simulink model "B64CostaTest"  (R2022a)
settings: Solver=VariableStepAuto  StartTime=0.0  StopTime=40  RelTol=1e-4  AbsTol=1e-4
values from neighbouring files (symbols this model uses):
  AinfK_h_B64a = -23    [B64.m]
  AinfK_h_B64s = -23    [B64.m]
  AinfK_p_B64a = 1.0    (= 1)    [B64.m]
  AinfK_p_B64s = 1.0    (= 1)    [B64.m]
  AinfK_s_B64a = 9.0    (= 9)    [B64.m]
  AinfK_s_B64s = 9.0    (= 9)    [B64.m]
  AinfKpp_h_B64s = -50    [B64.m]
  AinfKpp_p_B64s = 1.0    (= 1)    [B64.m]
  AinfKpp_s_B64s = 1.0    (= 1)    [B64.m]
  AinfNa_h_B64a = -37    [B64.m]
  AinfNa_h_B64s = -37    [B64.m]
  AinfNa_p_B64a = 1.0    (= 1)    [B64.m]
  AinfNa_p_B64s = 1.0    (= 1)    [B64.m]
  AinfNa_s_B64a = 5.0    (= 5)    [B64.m]
  AinfNa_s_B64s = 5.0    (= 5)    [B64.m]
  AinfNapp_h_B64s = -50    [B64.m]
  AinfNapp_p_B64s = 1.0    (= 1)    [B64.m]
  AinfNapp_s_B64s = 1.0    (= 1)    [B64.m]
  AK_B64a_0 = 0.5    [B64.m]
  AK_B64s_0 = 0.5    [B64.m]
  AKpp_B64s_0 = 0.5    [B64.m]
  ANa_B64a_0 = 0.5    [B64.m]
  ANa_B64s_0 = 0.5    [B64.m]
  ANapp_B64s_0 = 0.5    [B64.m]
  BinfNa_h_B64a = -43.0    (= -43)    [B64.m]
  BinfNa_h_B64s = -43.0    (= -43)    [B64.m]
  BinfNa_p_B64a = 1.0    (= 1)    [B64.m]
  BinfNa_p_B64s = 1.0    (= 1)    [B64.m]
  BinfNa_s_B64a = 5.0    (= 5)    [B64.m]
  BinfNa_s_B64s = 5.0    (= 5)    [B64.m]
  BNa_B64a_0 = 0.5    [B64.m]
  BNa_B64s_0 = 0.5    [B64.m]
  Cm_B64a = 0.01    [B64.m]
  Cm_B64s = 0.01    [B64.m]
  EK_B64a = -70    [B64.m]
  EK_B64s = -80    [B64.m]
  EKpp_B64s = -70    [B64.m]
  EL_B64a = -60    [B64.m]
  EL_B64s = -60    [B64.m]
  ENa_B64a = 30    [B64.m]
  ENa_B64s = 30    [B64.m]
  ENapp_B64s = 30    [B64.m]
  gec_B64a2B64s = 0.25    [B64.m]
  gec_B64s2B64a = 0.25    [B64.m]
  gK_B64a = 14    [B64.m]
  gK_B64s = 1.2    [B64.m]
  gKpp_B64s = 0.35    [B64.m]
  gL_B64a = 0.1    [B64.m]
  gL_B64s = 0.1    [B64.m]
  gNa_B64a = 25    [B64.m]
  gNa_B64s = 2.5    [B64.m]
  gNapp_B64s = 0.1    [B64.m]
  pK_B64a = 4    [B64.m]
  pK_B64s = 4    [B64.m]
  pKpp_B64s = 1    [B64.m]
  pNa_B64a = 3    [B64.m]
  pNa_B64s = 3    [B64.m]
  pNapp_B64s = 1    [B64.m]
  RK_B64a = 0    [B64.m]
  RK_B64s = 0    [B64.m]
  RKpp_B64s = 0    [B64.m]
  RL_B64a = 0    [B64.m]
  RL_B64s = 0    [B64.m]
  RNa_B64a = 0    [B64.m]
  RNa_B64s = 0    [B64.m]
  RNapp_B64s = 0    [B64.m]
  spikedur_B64a = 0.003    [B64.m]
  tAK_h_B64a = -8.0    (= -8)    [B64.m]
  tAK_h_B64s = -8.0    (= -8)    [B64.m]
  tAK_p_B64a = 1.0    (= 1)    [B64.m]
  tAK_p_B64s = 1.0    (= 1)    [B64.m]
  tAK_s_B64a = 10.0    (= 10)    [B64.m]
  tAK_s_B64s = 10.0    (= 10)    [B64.m]
  tAK_tmax_B64a = 0.04    [B64.m]
  tAK_tmax_B64s = 0.04    [B64.m]
  tAK_tmin_B64a = 0.004    [B64.m]
  tAK_tmin_B64s = 0.004    [B64.m]
  tAKpp_t_B64s = 4    [B64.m]
  tANa_h_B64a = -43    [B64.m]
  tANa_h_B64s = -43    [B64.m]
  tANa_p_B64a = 1.0    (= 1)    [B64.m]
  tANa_p_B64s = 1.0    (= 1)    [B64.m]
  tANa_s_B64a = 4.0    (= 4)    [B64.m]
  tANa_s_B64s = 4.0    (= 4)    [B64.m]
  tANa_tmax_B64a = 0.006    [B64.m]
  tANa_tmax_B64s = 0.006    [B64.m]
  tANa_tmin_B64a = 0.001    [B64.m]
  tANa_tmin_B64s = 0.001    [B64.m]
  tANapp_t_B64s = 0.1    [B64.m]
  tBNa_h_B64a = -38    [B64.m]
  tBNa_h_B64s = -38    [B64.m]
  tBNa_p_B64a = 1.0    (= 1)    [B64.m]
  tBNa_p_B64s = 1.0    (= 1)    [B64.m]
  tBNa_s_B64a = 10.0    (= 10)    [B64.m]
  tBNa_s_B64s = 10.0    (= 10)    [B64.m]
  tBNa_tmax_B64a = 0.02    [B64.m]
  tBNa_tmax_B64s = 0.02    [B64.m]
  tBNa_tmin_B64a = 0.005    [B64.m]
  tBNa_tmin_B64s = 0.005    [B64.m]
  V_B64a_0 = -60    [B64.m]
  V_B64s_0 = -60    [B64.m]
undefined symbols (not defined in the file or in its folder): Iapp
libraries: simulink x1
settings Model: Creator=liyan  LastModifiedBy=liyan

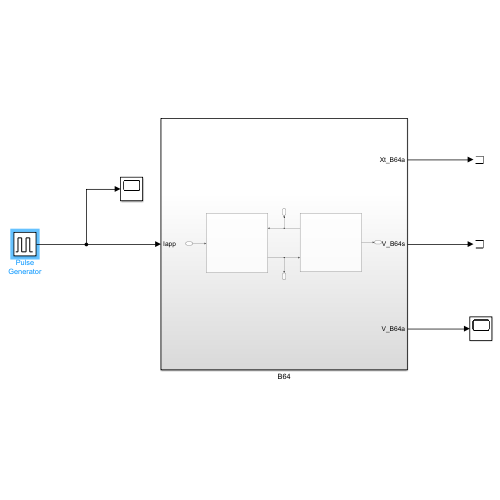
[thumbnail: Simulink's stored preview of the top-level diagram]
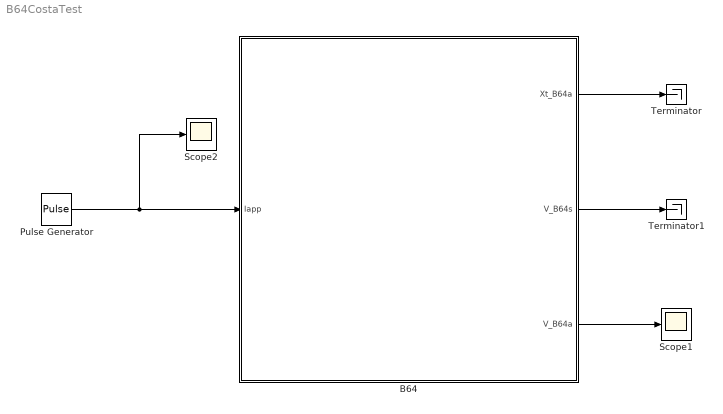
== system B64CostaTest ==
  B64 : Subsystem
  Pulse Generator : DiscretePulseGenerator  PulseType=Time based  Amplitude=Iapp  Period=40  PulseWidth=0.3/40*100  PhaseDelay=30
  Scope1 : Scope
  Scope2 : Scope
  Terminator : Terminator
  Terminator1 : Terminator
  wires:
  Pulse Generator/1 -> B64/1(Iapp), Scope2/1
  B64/2(V_B64s) -> Terminator1/1
  B64/3(V_B64a) -> Scope1/1
  B64/1(Xt_B64a) -> Terminator/1

== system B64CostaTest/B64 ==
  Iapp : Inport
  Axon : Subsystem
      settings: PortSchema="{\"entries\":[{\"content\":{\"sides\":[{\"content\":{\"connectorIds\":[\"In1\",\"Out2\"]},\"type\":\"ConnectorPlacement.EquallySpacedRectSide\",\"uuid\":\"40bd10fa-ed99-4b6a-86ee-aa667b2fa219\"},{\"content\":{\"connectorIds\":[\"Out1\"],\"side\":\"RIGHT\"},\"type\":\"ConnectorPlacement.EquallySpacedRectSide\",\"uuid\":\"a431bac5-795f-4390-8885-144606cfe2c6\"},{\"content\":{\"connectorIds\":[],\"side\":\"TOP\"},\"type\":\"ConnectorPlacement.EquallySpacedRectSide\",\"uuid\":\"7e20a892-1662-4491-8c8d-274d49de163b\"},{\"content\":{\"connectorIds\":[],\"side\":\"BOTTOM\"},\"type\":\"ConnectorPlacement.EquallySpacedRectSide\",\"uuid\":\"ab3dc877-3a3e-482a-aafe-64d6d0026420\"}]},\"type\":\"ConnectorPlacement.EquallySpacedConnector\",\"uuid\":\"01fbcc32-18b1-446e-a5b1-3660a779301b\"}],\"packageUris\":[\"http://schema.mathworks.com/mf0/Connector/R2020b\"],\"version\":\"1.0\"}"
  Soma : Subsystem
      settings: PortSchema="{\"entries\":[{\"content\":{\"sides\":[{\"content\":{\"connectorIds\":[\"In1\"]},\"type\":\"ConnectorPlacement.EquallySpacedRectSide\",\"uuid\":\"61f6e0bf-b055-4ffe-aeac-0536888a11b7\"},{\"content\":{\"connectorIds\":[\"Out1\",\"In2\"],\"side\":\"RIGHT\"},\"type\":\"ConnectorPlacement.EquallySpacedRectSide\",\"uuid\":\"fd31abd7-219d-468a-b386-105a5f18ecba\"},{\"content\":{\"connectorIds\":[],\"side\":\"TOP\"},\"type\":\"ConnectorPlacement.EquallySpacedRectSide\",\"uuid\":\"61248356-ebfa-4703-87fc-ac9a699c85cb\"},{\"content\":{\"connectorIds\":[],\"side\":\"BOTTOM\"},\"type\":\"ConnectorPlacement.EquallySpacedRectSide\",\"uuid\":\"824f436a-a50d-431e-bf8e-5e4435a63c06\"}]},\"type\":\"ConnectorPlacement.EquallySpacedConnector\",\"uuid\":\"04bfac00-4a5c-4c95-bc84-ba6035aba6c8\"}],\"packageUris\":[\"http://schema.mathworks.com/mf0/Connector/R2020b\"],\"version\":\"1.0\"}"
  Xt_B64a : Outport
  V_B64s : Outport  Port=2
  V_B64a : Outport  Port=3
  wires:
  Axon/2(V_B64a) -> V_B64a/1, Soma/2(V_B64a)
  Soma/1(V_B64s) -> V_B64s/1, Axon/1(V_B64s)
  Axon/1(Xt_B64a) -> Xt_B64a/1
  Iapp/1 -> Soma/1(Iapp)

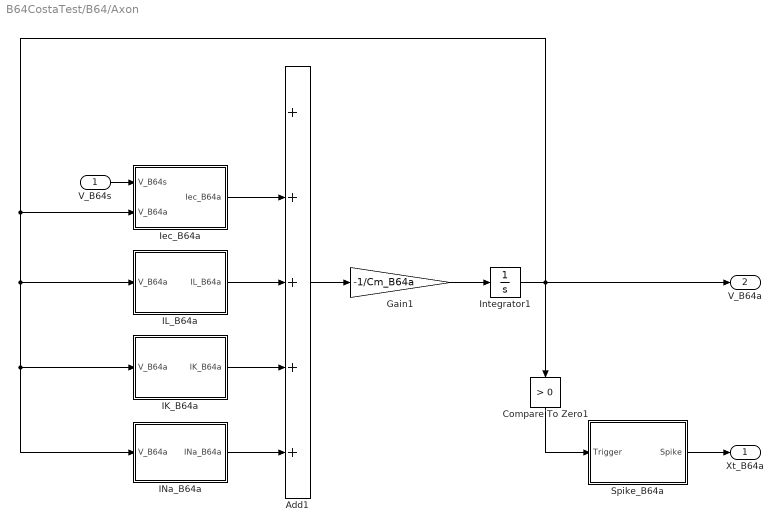
== system B64CostaTest/B64/Axon ==
  V_B64s : Inport
  Add1 : Sum  Inputs=+++++
  Compare To Zero1 : simulink/Logic and Bit Operations/Compare To Zero  relop=>  OutDataTypeStr=boolean
  Gain1 : Gain  Gain=-1/Cm_B64a
  IK_B64a : Subsystem
  IL_B64a : Subsystem
  INa_B64a : Subsystem
  Iec_B64a : Subsystem
  Integrator1 : Integrator  InitialCondition=V_B64a_0
  Spike_B64a : Subsystem
  Xt_B64a : Outport
  V_B64a : Outport  Port=2
  wires:
  Add1/1 -> Gain1/1
  Gain1/1 -> Integrator1/1
  Integrator1/1 -> Iec_B64a/2(V_B64a), IL_B64a/1(V_B64a), IK_B64a/1(V_B64a), INa_B64a/1(V_B64a), Compare To Zero1/1, V_B64a/1
  V_B64s/1 -> Iec_B64a/1(V_B64s)
  Compare To Zero1/1 -> Spike_B64a/1(Trigger)
  Spike_B64a/1(Spike) -> Xt_B64a/1
  INa_B64a/1(INa_B64a) -> Add1/5
  IK_B64a/1(IK_B64a) -> Add1/4
  IL_B64a/1(IL_B64a) -> Add1/3
  Iec_B64a/1(Iec_B64a) -> Add1/2

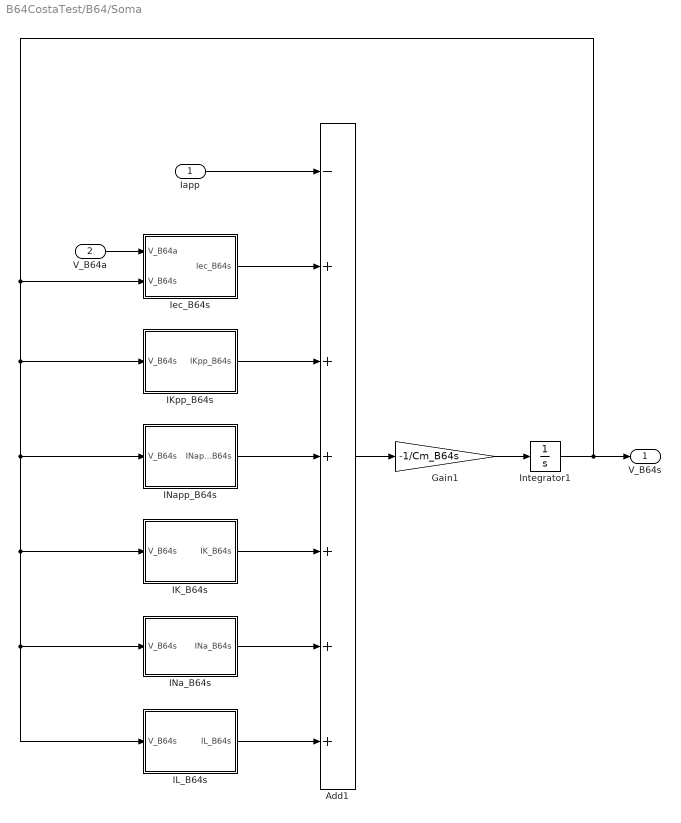
== system B64CostaTest/B64/Soma ==
  Iapp : Inport
  V_B64a : Inport  Port=2
  Add1 : Sum  Inputs=-++++++
  Gain1 : Gain  Gain=-1/Cm_B64s
  IK_B64s : Subsystem
  IKpp_B64s : Subsystem
  IL_B64s : Subsystem
  INa_B64s : Subsystem
  INapp_B64s : Subsystem
  Iec_B64s : Subsystem
  Integrator1 : Integrator  InitialCondition=V_B64s_0
  V_B64s : Outport
  wires:
  Add1/1 -> Gain1/1
  Gain1/1 -> Integrator1/1
  V_B64a/1 -> Iec_B64s/1(V_B64a)
  IL_B64s/1(IL_B64s) -> Add1/7
  INa_B64s/1(INa_B64s) -> Add1/6
  IK_B64s/1(IK_B64s) -> Add1/5
  INapp_B64s/1(INapp_B64s) -> Add1/4
  IKpp_B64s/1(IKpp_B64s) -> Add1/3
  Iec_B64s/1(Iec_B64s) -> Add1/2
  Integrator1/1 -> V_B64s/1, IKpp_B64s/1(V_B64s), INapp_B64s/1(V_B64s), IK_B64s/1(V_B64s), INa_B64s/1(V_B64s), IL_B64s/1(V_B64s), Iec_B64s/2(V_B64s)
  Iapp/1 -> Add1/1

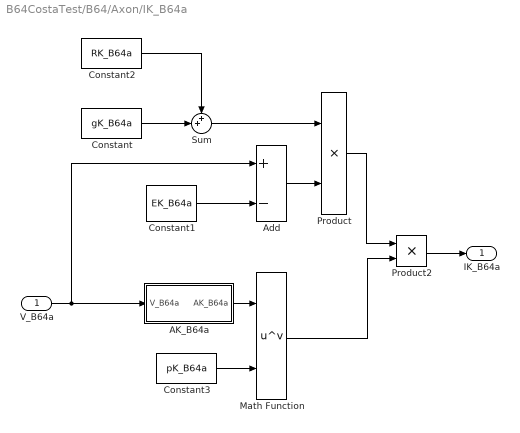
== system B64CostaTest/B64/Axon/IK_B64a ==
  V_B64a : Inport
  AK_B64a : Subsystem
  Add : Sum  Inputs=+-
  Constant : Constant  Value=gK_B64a
  Constant1 : Constant  Value=EK_B64a
  Constant2 : Constant  Value=RK_B64a
  Constant3 : Constant  Value=pK_B64a
  Math Function : Math  Operator=pow
  Product : Product
  Product2 : Product
  Sum : Sum  Inputs=++|
  IK_B64a : Outport
  wires:
  Add/1 -> Product/2
  Constant1/1 -> Add/2
  V_B64a/1 -> AK_B64a/1(V_B64a), Add/1
  Product/1 -> Product2/1
  Math Function/1 -> Product2/2
  Product2/1 -> IK_B64a/1
  Constant/1 -> Sum/2
  Sum/1 -> Product/1
  Constant2/1 -> Sum/1
  AK_B64a/1(AK_B64a) -> Math Function/1
  Constant3/1 -> Math Function/2

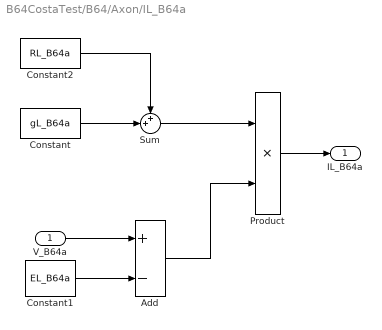
== system B64CostaTest/B64/Axon/IL_B64a ==
  V_B64a : Inport
  Add : Sum  Inputs=+-
  Constant : Constant  Value=gL_B64a
  Constant1 : Constant  Value=EL_B64a
  Constant2 : Constant  Value=RL_B64a
  Product : Product
  Sum : Sum  Inputs=++|
  IL_B64a : Outport
  wires:
  Constant1/1 -> Add/2
  V_B64a/1 -> Add/1
  Constant2/1 -> Sum/1
  Sum/1 -> Product/1
  Constant/1 -> Sum/2
  Add/1 -> Product/2
  Product/1 -> IL_B64a/1

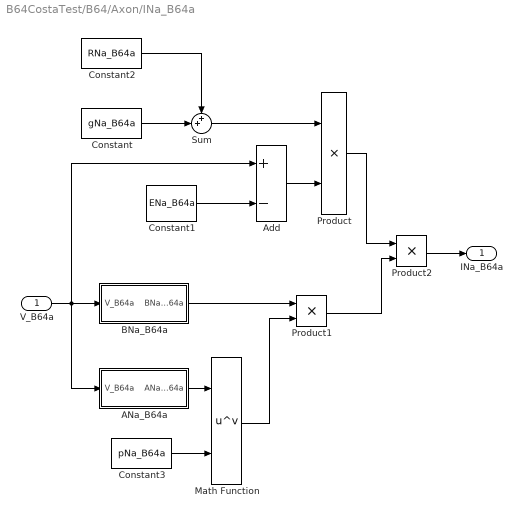
== system B64CostaTest/B64/Axon/INa_B64a ==
  V_B64a : Inport
  ANa_B64a : Subsystem
  Add : Sum  Inputs=+-
  BNa_B64a : Subsystem
  Constant : Constant  Value=gNa_B64a
  Constant1 : Constant  Value=ENa_B64a
  Constant2 : Constant  Value=RNa_B64a
  Constant3 : Constant  Value=pNa_B64a
  Math Function : Math  Operator=pow
  Product : Product
  Product1 : Product
  Product2 : Product
  Sum : Sum  Inputs=++|
  INa_B64a : Outport
  wires:
  Add/1 -> Product/2
  Constant1/1 -> Add/2
  V_B64a/1 -> ANa_B64a/1(V_B64a), BNa_B64a/1(V_B64a), Add/1
  Product/1 -> Product2/1
  Product1/1 -> Product2/2
  Product2/1 -> INa_B64a/1
  Constant/1 -> Sum/2
  Sum/1 -> Product/1
  Constant2/1 -> Sum/1
  ANa_B64a/1(ANa_B64a) -> Math Function/1
  Constant3/1 -> Math Function/2
  BNa_B64a/1(BNa_B64a) -> Product1/1
  Math Function/1 -> Product1/2

== system B64CostaTest/B64/Axon/Iec_B64a ==
  V_B64s : Inport
  V_B64a : Inport  Port=2
  Add : Sum  Inputs=-+
  Gain : Gain  Gain=gec_B64s2B64a
  Iec_B64a : Outport
  wires:
  Add/1 -> Gain/1
  V_B64s/1 -> Add/1
  V_B64a/1 -> Add/2
  Gain/1 -> Iec_B64a/1

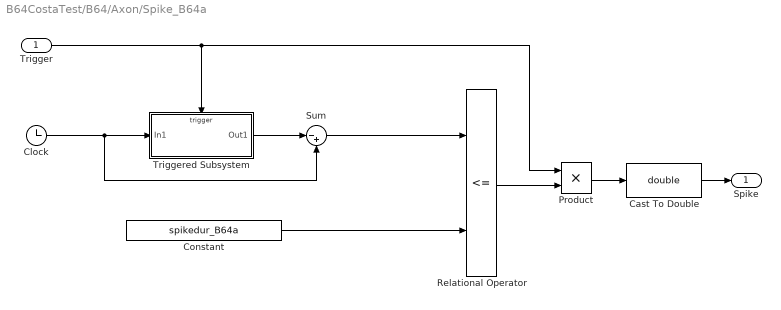
== system B64CostaTest/B64/Axon/Spike_B64a ==
  Trigger : Inport
  Cast To Double : DataTypeConversion  OutDataTypeStr=double  SaturateOnIntegerOverflow=off  RndMeth=Floor
  Clock : Clock
  Constant : Constant  Value=spikedur_B64a
  Product : Product
  Relational Operator : RelationalOperator  Operator=<=  OutDataTypeStr=boolean  RndMeth=Simplest  InputSameDT=off
  Sum : Sum  Inputs=|-+
  Triggered Subsystem : Subsystem  TreatAsAtomicUnit=on
  Spike : Outport
  wires:
  Clock/1 -> Sum/2, Triggered Subsystem/1(In1)
  Triggered Subsystem/1(Out1) -> Sum/1
  Constant/1 -> Relational Operator/2
  Trigger/1 -> Triggered Subsystem/Trigger, Product/1
  Sum/1 -> Relational Operator/1
  Relational Operator/1 -> Product/2
  Cast To Double/1 -> Spike/1
  Product/1 -> Cast To Double/1

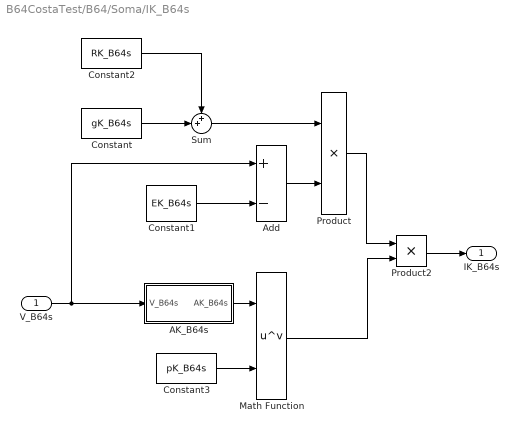
== system B64CostaTest/B64/Soma/IK_B64s ==
  V_B64s : Inport
  AK_B64s : Subsystem
  Add : Sum  Inputs=+-
  Constant : Constant  Value=gK_B64s
  Constant1 : Constant  Value=EK_B64s
  Constant2 : Constant  Value=RK_B64s
  Constant3 : Constant  Value=pK_B64s
  Math Function : Math  Operator=pow
  Product : Product
  Product2 : Product
  Sum : Sum  Inputs=++|
  IK_B64s : Outport
  wires:
  Add/1 -> Product/2
  Constant1/1 -> Add/2
  V_B64s/1 -> AK_B64s/1(V_B64s), Add/1
  Product/1 -> Product2/1
  Math Function/1 -> Product2/2
  Product2/1 -> IK_B64s/1
  Constant/1 -> Sum/2
  Sum/1 -> Product/1
  Constant2/1 -> Sum/1
  AK_B64s/1(AK_B64s) -> Math Function/1
  Constant3/1 -> Math Function/2

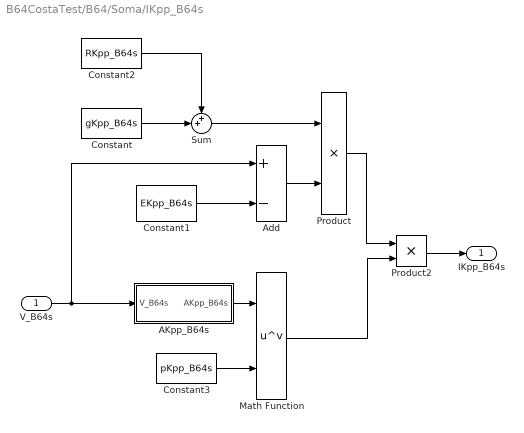
== system B64CostaTest/B64/Soma/IKpp_B64s ==
  V_B64s : Inport
  AKpp_B64s : Subsystem
  Add : Sum  Inputs=+-
  Constant : Constant  Value=gKpp_B64s
  Constant1 : Constant  Value=EKpp_B64s
  Constant2 : Constant  Value=RKpp_B64s
  Constant3 : Constant  Value=pKpp_B64s
  Math Function : Math  Operator=pow
  Product : Product
  Product2 : Product
  Sum : Sum  Inputs=++|
  IKpp_B64s : Outport
  wires:
  Add/1 -> Product/2
  Constant1/1 -> Add/2
  V_B64s/1 -> AKpp_B64s/1(V_B64s), Add/1
  Product/1 -> Product2/1
  Math Function/1 -> Product2/2
  Product2/1 -> IKpp_B64s/1
  Constant/1 -> Sum/2
  Sum/1 -> Product/1
  Constant2/1 -> Sum/1
  AKpp_B64s/1(AKpp_B64s) -> Math Function/1
  Constant3/1 -> Math Function/2

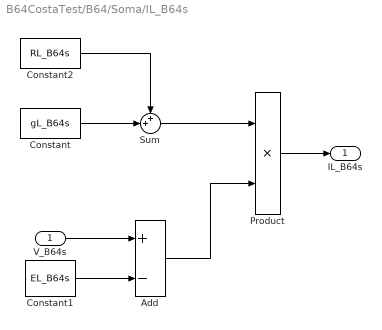
== system B64CostaTest/B64/Soma/IL_B64s ==
  V_B64s : Inport
  Add : Sum  Inputs=+-
  Constant : Constant  Value=gL_B64s
  Constant1 : Constant  Value=EL_B64s
  Constant2 : Constant  Value=RL_B64s
  Product : Product
  Sum : Sum  Inputs=++|
  IL_B64s : Outport
  wires:
  Constant1/1 -> Add/2
  V_B64s/1 -> Add/1
  Constant2/1 -> Sum/1
  Sum/1 -> Product/1
  Constant/1 -> Sum/2
  Add/1 -> Product/2
  Product/1 -> IL_B64s/1

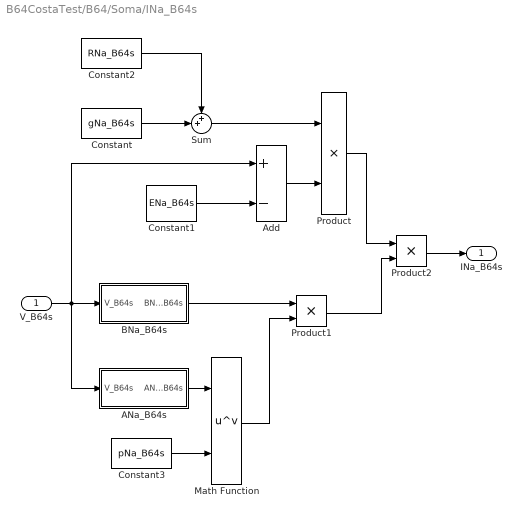
== system B64CostaTest/B64/Soma/INa_B64s ==
  V_B64s : Inport
  ANa_B64s : Subsystem
  Add : Sum  Inputs=+-
  BNa_B64s : Subsystem
  Constant : Constant  Value=gNa_B64s
  Constant1 : Constant  Value=ENa_B64s
  Constant2 : Constant  Value=RNa_B64s
  Constant3 : Constant  Value=pNa_B64s
  Math Function : Math  Operator=pow
  Product : Product
  Product1 : Product
  Product2 : Product
  Sum : Sum  Inputs=++|
  INa_B64s : Outport
  wires:
  Add/1 -> Product/2
  Constant1/1 -> Add/2
  V_B64s/1 -> ANa_B64s/1(V_B64s), BNa_B64s/1(V_B64s), Add/1
  Product/1 -> Product2/1
  Product1/1 -> Product2/2
  Product2/1 -> INa_B64s/1
  Constant/1 -> Sum/2
  Sum/1 -> Product/1
  Constant2/1 -> Sum/1
  ANa_B64s/1(ANa_B64s) -> Math Function/1
  Constant3/1 -> Math Function/2
  BNa_B64s/1(BNa_B64s) -> Product1/1
  Math Function/1 -> Product1/2

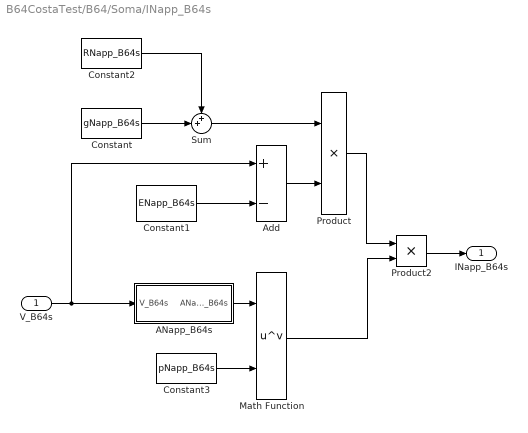
== system B64CostaTest/B64/Soma/INapp_B64s ==
  V_B64s : Inport
  ANapp_B64s : Subsystem
  Add : Sum  Inputs=+-
  Constant : Constant  Value=gNapp_B64s
  Constant1 : Constant  Value=ENapp_B64s
  Constant2 : Constant  Value=RNapp_B64s
  Constant3 : Constant  Value=pNapp_B64s
  Math Function : Math  Operator=pow
  Product : Product
  Product2 : Product
  Sum : Sum  Inputs=++|
  INapp_B64s : Outport
  wires:
  Add/1 -> Product/2
  Constant1/1 -> Add/2
  V_B64s/1 -> ANapp_B64s/1(V_B64s), Add/1
  Product/1 -> Product2/1
  Math Function/1 -> Product2/2
  Product2/1 -> INapp_B64s/1
  Constant/1 -> Sum/2
  Sum/1 -> Product/1
  Constant2/1 -> Sum/1
  ANapp_B64s/1(ANapp_B64s) -> Math Function/1
  Constant3/1 -> Math Function/2

== system B64CostaTest/B64/Soma/Iec_B64s ==
  V_B64a : Inport
  V_B64s : Inport  Port=2
  Add : Sum  Inputs=-+
  Gain : Gain  Gain=gec_B64a2B64s
  Iec_B64s : Outport
  wires:
  Add/1 -> Gain/1
  V_B64a/1 -> Add/1
  V_B64s/1 -> Add/2
  Gain/1 -> Iec_B64s/1

== system B64CostaTest/B64/Axon/IK_B64a/AK_B64a ==
  V_B64a : Inport
  AKinf_B64a : MATLABFcn  MATLABFcn=1/(1 + exp((AinfK_h_B64a - u(1))/AinfK_s_B64a))^AinfK_p_B64a
  Add1 : Sum  Inputs=-+
  Divide : Product  Inputs=*/
  Integrator1 : Integrator  InitialCondition=AK_B64a_0
  tauAK_B64a : MATLABFcn  MATLABFcn=tAK_tmin_B64a + (tAK_tmax_B64a - tAK_tmin_B64a)/(1 + exp((u(1) - tAK_h_B64a)/tAK_s_B64a))^tAK_p_B64a
  AK_B64a : Outport
  wires:
  tauAK_B64a/1 -> Divide/2
  Divide/1 -> Integrator1/1
  V_B64a/1 -> tauAK_B64a/1, AKinf_B64a/1
  Integrator1/1 -> Add1/1, AK_B64a/1
  Add1/1 -> Divide/1
  AKinf_B64a/1 -> Add1/2

== system B64CostaTest/B64/Axon/INa_B64a/ANa_B64a ==
  V_B64a : Inport
  ANainf_B64a : MATLABFcn  MATLABFcn=1/(1 + exp((AinfNa_h_B64a - u(1))/AinfNa_s_B64a))^AinfNa_p_B64a
  Add1 : Sum  Inputs=-+
  Divide : Product  Inputs=*/
  Integrator1 : Integrator  InitialCondition=ANa_B64a_0
  tauANa_B64a : MATLABFcn  MATLABFcn=tANa_tmin_B64a + (tANa_tmax_B64a - tANa_tmin_B64a)/(1 + exp((u(1) - tANa_h_B64a)/tANa_s_B64a))^tANa_p_B64a
  ANa_B64a : Outport
  wires:
  tauANa_B64a/1 -> Divide/2
  Divide/1 -> Integrator1/1
  V_B64a/1 -> tauANa_B64a/1, ANainf_B64a/1
  Integrator1/1 -> Add1/1, ANa_B64a/1
  Add1/1 -> Divide/1
  ANainf_B64a/1 -> Add1/2

== system B64CostaTest/B64/Axon/INa_B64a/BNa_B64a ==
  V_B64a : Inport
  Add1 : Sum  Inputs=-+
  BNainf_B64a : MATLABFcn  MATLABFcn=1/(1 + exp((u(1) - BinfNa_h_B64a)/BinfNa_s_B64a))^BinfNa_p_B64a
  Divide : Product  Inputs=*/
  Integrator1 : Integrator  InitialCondition=BNa_B64a_0
  tauBNa_B64a : MATLABFcn  MATLABFcn=tBNa_tmin_B64a + (tBNa_tmax_B64a - tBNa_tmin_B64a)/(1 + exp((u(1) - tBNa_h_B64a)/tBNa_s_B64a))^tBNa_p_B64a
  BNa_B64a : Outport
  wires:
  tauBNa_B64a/1 -> Divide/2
  Divide/1 -> Integrator1/1
  V_B64a/1 -> tauBNa_B64a/1, BNainf_B64a/1
  Integrator1/1 -> Add1/1, BNa_B64a/1
  Add1/1 -> Divide/1
  BNainf_B64a/1 -> Add1/2

== system B64CostaTest/B64/Axon/Spike_B64a/Triggered Subsystem ==
  In1 : Inport
  Trigger : TriggerPort  VariantControl=Variant
  Out1 : Outport
  wires:
  In1/1 -> Out1/1

== system B64CostaTest/B64/Soma/IK_B64s/AK_B64s ==
  V_B64s : Inport
  AKinf_B64s : MATLABFcn  MATLABFcn=1/(1 + exp((AinfK_h_B64s - u(1))/AinfK_s_B64s))^AinfK_p_B64s
  Add1 : Sum  Inputs=-+
  Divide : Product  Inputs=*/
  Integrator1 : Integrator  InitialCondition=AK_B64s_0
  tauAK_B64s : MATLABFcn  MATLABFcn=tAK_tmin_B64s + (tAK_tmax_B64s - tAK_tmin_B64s)/(1 + exp((u(1) - tAK_h_B64s)/tAK_s_B64s))^tAK_p_B64s
  AK_B64s : Outport
  wires:
  tauAK_B64s/1 -> Divide/2
  Divide/1 -> Integrator1/1
  V_B64s/1 -> tauAK_B64s/1, AKinf_B64s/1
  Integrator1/1 -> Add1/1, AK_B64s/1
  Add1/1 -> Divide/1
  AKinf_B64s/1 -> Add1/2

== system B64CostaTest/B64/Soma/IKpp_B64s/AKpp_B64s ==
  V_B64s : Inport
  AKppinf_B64s : MATLABFcn  MATLABFcn=1/(1 + exp((AinfKpp_h_B64s - u(1))/AinfKpp_s_B64s))^AinfKpp_p_B64s
  Add1 : Sum  Inputs=-+
  Constant : Constant  Value=tAKpp_t_B64s
  Divide : Product  Inputs=*/
  Integrator1 : Integrator  InitialCondition=AKpp_B64s_0
  AKpp_B64s : Outport
  wires:
  Constant/1 -> Divide/2
  Divide/1 -> Integrator1/1
  V_B64s/1 -> AKppinf_B64s/1
  Integrator1/1 -> Add1/1, AKpp_B64s/1
  Add1/1 -> Divide/1
  AKppinf_B64s/1 -> Add1/2

== system B64CostaTest/B64/Soma/INa_B64s/ANa_B64s ==
  V_B64s : Inport
  ANainf_B64s : MATLABFcn  MATLABFcn=1/(1 + exp((AinfNa_h_B64s - u(1))/AinfNa_s_B64s))^AinfNa_p_B64s
  Add1 : Sum  Inputs=-+
  Divide : Product  Inputs=*/
  Integrator1 : Integrator  InitialCondition=ANa_B64s_0
  tauANa_B64s : MATLABFcn  MATLABFcn=tANa_tmin_B64s + (tANa_tmax_B64s - tANa_tmin_B64s)/(1 + exp((u(1) - tANa_h_B64s)/tANa_s_B64s))^tANa_p_B64s
  ANa_B64s : Outport
  wires:
  tauANa_B64s/1 -> Divide/2
  Divide/1 -> Integrator1/1
  V_B64s/1 -> tauANa_B64s/1, ANainf_B64s/1
  Integrator1/1 -> Add1/1, ANa_B64s/1
  Add1/1 -> Divide/1
  ANainf_B64s/1 -> Add1/2

== system B64CostaTest/B64/Soma/INa_B64s/BNa_B64s ==
  V_B64s : Inport
  Add1 : Sum  Inputs=-+
  BNainf_B64s : MATLABFcn  MATLABFcn=1/(1 + exp((u(1) - BinfNa_h_B64s)/BinfNa_s_B64s))^BinfNa_p_B64s
  Divide : Product  Inputs=*/
  Integrator1 : Integrator  InitialCondition=BNa_B64s_0
  tauBNa_B64s : MATLABFcn  MATLABFcn=tBNa_tmin_B64s + (tBNa_tmax_B64s - tBNa_tmin_B64s)/(1 + exp((u(1) - tBNa_h_B64s)/tBNa_s_B64s))^tBNa_p_B64s
  BNa_B64s : Outport
  wires:
  tauBNa_B64s/1 -> Divide/2
  Divide/1 -> Integrator1/1
  V_B64s/1 -> tauBNa_B64s/1, BNainf_B64s/1
  Integrator1/1 -> Add1/1, BNa_B64s/1
  Add1/1 -> Divide/1
  BNainf_B64s/1 -> Add1/2

== system B64CostaTest/B64/Soma/INapp_B64s/ANapp_B64s ==
  V_B64s : Inport
  ANappinf_B64s : MATLABFcn  MATLABFcn=1/(1 + exp((AinfNapp_h_B64s - u(1))/AinfNapp_s_B64s))^AinfNapp_p_B64s
  Add1 : Sum  Inputs=-+
  Constant : Constant  Value=tANapp_t_B64s
  Divide : Product  Inputs=*/
  Integrator1 : Integrator  InitialCondition=ANapp_B64s_0
  ANapp_B64s : Outport
  wires:
  Constant/1 -> Divide/2
  Divide/1 -> Integrator1/1
  V_B64s/1 -> ANappinf_B64s/1
  Integrator1/1 -> Add1/1, ANapp_B64s/1
  Add1/1 -> Divide/1
  ANappinf_B64s/1 -> Add1/2
